simulink model "single_module"  (R2018a)
settings: Solver=FixedStepDiscrete  StartTime=0.0  StopTime=Tfinal  FixedStep=SampleTime  RelTol=1e-3
values from neighbouring files (symbols this model uses):
  C1A = 5e-6    (= 5e-06)    [capacitor_A.m]    (also in impedance_phA.m; param_single_module_parasitic.m; trial_capacitor_response.m)
  C1B = 5e-6    (= 5e-06)    [capacitor_A.m]    (also in impedance_phA.m; param_single_module_parasitic.m; trial_capacitor_response.m)
  C1C = 5e-6    (= 5e-06)    [capacitor_A.m]    (also in impedance_phA.m; param_single_module_parasitic.m; trial_capacitor_response.m)
  ESLA = 19e-9    (= 1.9e-08)    [capacitor_A.m]    (also in impedance_phA.m; param_single_module_parasitic.m; trial_capacitor_response.m)
  ESLB = 19e-9    (= 1.9e-08)    [capacitor_A.m]    (also in impedance_phA.m; param_single_module_parasitic.m; trial_capacitor_response.m)
  ESLC = 19e-9    (= 1.9e-08)    [capacitor_A.m]    (also in impedance_phA.m; param_single_module_parasitic.m; trial_capacitor_response.m)
  ESRA = 21.1e-3    (= 0.0211)    [impedance_phA.m]    (also in param_single_module_parasitic.m)
  ESRB = 21.1e-3    (= 0.0211)    [impedance_phA.m]    (also in param_single_module_parasitic.m)
  ESRC = 21.1e-3    (= 0.0211)    [impedance_phA.m]    (also in param_single_module_parasitic.m)
  ffund = 50    [param_single_module_parasitic.m]
  LABBot = 10.20e-9    (= 1.02e-08)    [capacitor_A.m]    (also in impedance_phA.m; param_single_module_parasitic.m; trial_capacitor_response.m)
  LABot = 20.25e-9    (= 2.025e-08)    [capacitor_A.m]    (also in impedance_phA.m; param_single_module_parasitic.m; trial_capacitor_response.m)
  LABTop = 18.30e-9    (= 1.83e-08)    [capacitor_A.m]    (also in impedance_phA.m; param_single_module_parasitic.m; trial_capacitor_response.m)
  LAMid = 01.30e-9    (= 1.3e-09)    [capacitor_A.m]    (also in impedance_phA.m; param_single_module_parasitic.m; trial_capacitor_response.m)
  LATop = 03.40e-9    (= 3.4e-09)    [capacitor_A.m]    (also in impedance_phA.m; param_single_module_parasitic.m; trial_capacitor_response.m)
  LBBot = 20.38e-9    (= 2.038e-08)    [capacitor_A.m]    (also in impedance_phA.m; param_single_module_parasitic.m; trial_capacitor_response.m)
  LBCBot = 11.14e-9    (= 1.114e-08)    [capacitor_A.m]    (also in impedance_phA.m; param_single_module_parasitic.m; trial_capacitor_response.m)
  LBCTop = 21.84e-9    (= 2.184e-08)    [capacitor_A.m]    (also in impedance_phA.m; param_single_module_parasitic.m; trial_capacitor_response.m)
  LBMid = 01.30e-9    (= 1.3e-09)    [capacitor_A.m]    (also in impedance_phA.m; param_single_module_parasitic.m; trial_capacitor_response.m)
  LBTop = 03.38e-9    (= 3.38e-09)    [capacitor_A.m]    (also in impedance_phA.m; param_single_module_parasitic.m; trial_capacitor_response.m)
  LCBot = 20.94e-9    (= 2.094e-08)    [capacitor_A.m]    (also in impedance_phA.m; param_single_module_parasitic.m; trial_capacitor_response.m)
  LCMid = 01.30e-9    (= 1.3e-09)    [capacitor_A.m]    (also in impedance_phA.m; param_single_module_parasitic.m; trial_capacitor_response.m)
  LCTop = 03.41e-9    (= 3.41e-09)    [capacitor_A.m]    (also in impedance_phA.m; param_single_module_parasitic.m; trial_capacitor_response.m)
  Lin = 1e-4    (= 0.0001)    [capacitor_A.m]    (also in impedance_phA.m = 1e-06; param_single_module_parasitic.m = 1e-06; trial_capacitor_response.m)
  Lload1 = Xload1/(2*pi*ffund)    [param_single_module_parasitic.m]
  ModulationIndex1 = 0.9    [param_single_module_parasitic.m]
  Module1Phase = 0    [param_single_module_parasitic.m]
  Rin = 20    [capacitor_A.m]    (also in impedance_phA.m = 0.1; param_single_module_parasitic.m = 0.1; trial_capacitor_response.m = 50)
  Rload1 = Z1*PF    [param_single_module_parasitic.m]
  SampleTime = 1e-8    (= 1e-08)    [param_single_module_parasitic.m]
  Vin = Vdc + Idc*Rin    (= 270.740740741)    [param_single_module_parasitic.m]
libraries: powerlib x45, simulink x6, powerlib_meascontrol x1
settings Model: Creator=enes_  LastModifiedBy=enes_

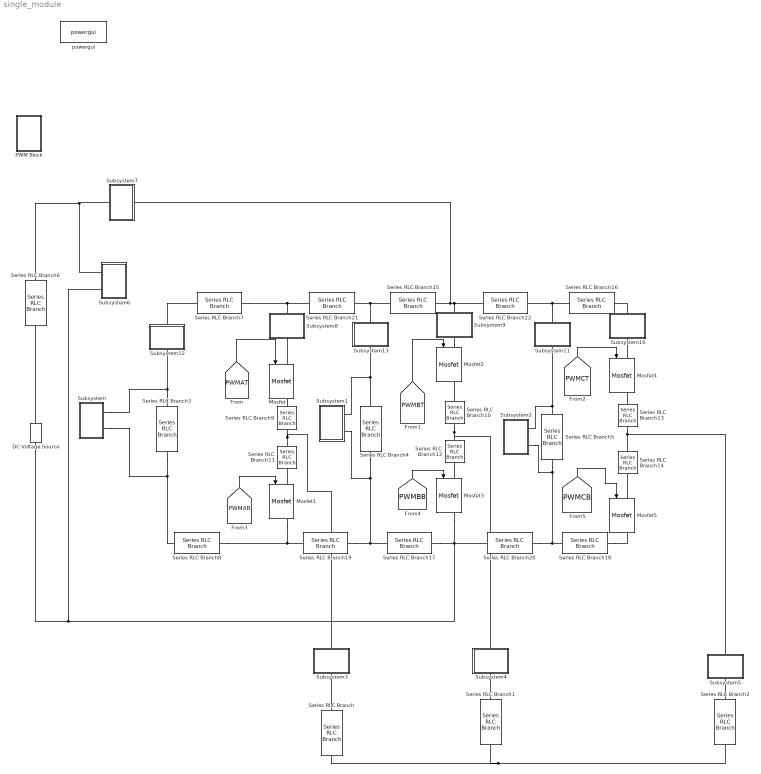
== system single_module ==
  DC Voltage Source : powerlib/Electrical Sources/DC Voltage Source  Amplitude=Vin  Measurements=None
  Mosfet{,1..5} (6 alike) : powerlib/Power Electronics/Mosfet  Ron=0.1  Lon=0  Rd=0.01  Vfd=0  IC=0  Rs=1e5  Cs=inf  Measurements=on
  PWM Block : Subsystem
  Series RLC Branch : powerlib/Elements/Series RLC Branch  LConnTagsString=__new0  RConnTagsString=__new0  BranchType=RL  Resistance=Rload1  Inductance=Lload1  SetiL0=off  InitialCurrent=0  Capacitance=1e-6  Setx0=off  InitialVoltage=0  Measurements=None
  Series RLC Branch1 : powerlib/Elements/Series RLC Branch  LConnTagsString=__new0  RConnTagsString=__new0  BranchType=RL  Resistance=Rload1  Inductance=Lload1  SetiL0=off  InitialCurrent=0  Capacitance=1e-6  Setx0=off  InitialVoltage=0  Measurements=None
  Series RLC Branch10 : powerlib/Elements/Series RLC Branch  LConnTagsString=__new0  RConnTagsString=__new0  BranchType=L  Resistance=1  Inductance=LBMid/2  SetiL0=off  InitialCurrent=0  Capacitance=1e-6  Setx0=off  InitialVoltage=0  Measurements=None
  Series RLC Branch11 : powerlib/Elements/Series RLC Branch  LConnTagsString=__new0  RConnTagsString=__new0  BranchType=L  Resistance=1  Inductance=LAMid/2  SetiL0=off  InitialCurrent=0  Capacitance=1e-6  Setx0=off  InitialVoltage=0  Measurements=None
  Series RLC Branch12 : powerlib/Elements/Series RLC Branch  LConnTagsString=__new0  RConnTagsString=__new0  BranchType=L  Resistance=1  Inductance=LBMid/2  SetiL0=off  InitialCurrent=0  Capacitance=1e-6  Setx0=off  InitialVoltage=0  Measurements=None
  Series RLC Branch13 : powerlib/Elements/Series RLC Branch  LConnTagsString=__new0  RConnTagsString=__new0  BranchType=L  Resistance=1  Inductance=LCMid/2  SetiL0=off  InitialCurrent=0  Capacitance=1e-6  Setx0=off  InitialVoltage=0  Measurements=None
  Series RLC Branch14 : powerlib/Elements/Series RLC Branch  LConnTagsString=__new0  RConnTagsString=__new0  BranchType=L  Resistance=1  Inductance=LCMid/2  SetiL0=off  InitialCurrent=0  Capacitance=1e-6  Setx0=off  InitialVoltage=0  Measurements=None
  Series RLC Branch15 : powerlib/Elements/Series RLC Branch  LConnTagsString=__new0  RConnTagsString=__new0  BranchType=L  Resistance=1  Inductance=LBTop  SetiL0=off  InitialCurrent=0  Capacitance=1e-6  Setx0=off  InitialVoltage=0  Measurements=None
  Series RLC Branch16 : powerlib/Elements/Series RLC Branch  LConnTagsString=__new0  RConnTagsString=__new0  BranchType=L  Resistance=1  Inductance=LCTop  SetiL0=off  InitialCurrent=0  Capacitance=1e-6  Setx0=off  InitialVoltage=0  Measurements=None
  Series RLC Branch17 : powerlib/Elements/Series RLC Branch  LConnTagsString=__new0  RConnTagsString=__new0  BranchType=L  Resistance=1  Inductance=LBBot  SetiL0=off  InitialCurrent=0  Capacitance=1e-6  Setx0=off  InitialVoltage=0  Measurements=None
  Series RLC Branch18 : powerlib/Elements/Series RLC Branch  LConnTagsString=__new0  RConnTagsString=__new0  BranchType=L  Resistance=1  Inductance=LCBot  SetiL0=off  InitialCurrent=0  Capacitance=1e-6  Setx0=off  InitialVoltage=0  Measurements=None
  Series RLC Branch19 : powerlib/Elements/Series RLC Branch  LConnTagsString=__new0  RConnTagsString=__new0  BranchType=L  Resistance=1  Inductance=LABBot  SetiL0=off  InitialCurrent=0  Capacitance=1e-6  Setx0=off  InitialVoltage=0  Measurements=None
  Series RLC Branch2 : powerlib/Elements/Series RLC Branch  LConnTagsString=__new0  RConnTagsString=__new0  BranchType=RL  Resistance=Rload1  Inductance=Lload1  SetiL0=off  InitialCurrent=0  Capacitance=1e-6  Setx0=off  InitialVoltage=0  Measurements=None
  Series RLC Branch20 : powerlib/Elements/Series RLC Branch  LConnTagsString=__new0  RConnTagsString=__new0  BranchType=L  Resistance=1  Inductance=LBCBot  SetiL0=off  InitialCurrent=0  Capacitance=1e-6  Setx0=off  InitialVoltage=0  Measurements=None
  Series RLC Branch21 : powerlib/Elements/Series RLC Branch  LConnTagsString=__new0  RConnTagsString=__new0  BranchType=L  Resistance=1  Inductance=LABTop  SetiL0=off  InitialCurrent=0  Capacitance=1e-6  Setx0=off  InitialVoltage=0  Measurements=None
  Series RLC Branch22 : powerlib/Elements/Series RLC Branch  LConnTagsString=__new0  RConnTagsString=__new0  BranchType=L  Resistance=1  Inductance=LBCTop  SetiL0=off  InitialCurrent=0  Capacitance=1e-6  Setx0=off  InitialVoltage=0  Measurements=None
  Series RLC Branch3 : powerlib/Elements/Series RLC Branch  LConnTagsString=__new0  RConnTagsString=__new0  BranchType=RLC  Resistance=ESRA  Inductance=ESLA  SetiL0=off  InitialCurrent=0  Capacitance=C1A  Setx0=off  InitialVoltage=0  Measurements=None
  Series RLC Branch4 : powerlib/Elements/Series RLC Branch  LConnTagsString=__new0  RConnTagsString=__new0  BranchType=RLC  Resistance=ESRB  Inductance=ESLB  SetiL0=off  InitialCurrent=0  Capacitance=C1B  Setx0=off  InitialVoltage=0  Measurements=None
  Series RLC Branch5 : powerlib/Elements/Series RLC Branch  LConnTagsString=__new0  RConnTagsString=__new0  BranchType=RLC  Resistance=ESRC  Inductance=ESLC  SetiL0=off  InitialCurrent=0  Capacitance=C1C  Setx0=off  InitialVoltage=0  Measurements=None
  Series RLC Branch6 : powerlib/Elements/Series RLC Branch  LConnTagsString=__new0  RConnTagsString=__new0  BranchType=RL  Resistance=Rin  Inductance=Lin  SetiL0=off  InitialCurrent=0  Capacitance=C1A  Setx0=off  InitialVoltage=0  Measurements=None
  Series RLC Branch7 : powerlib/Elements/Series RLC Branch  LConnTagsString=__new0  RConnTagsString=__new0  BranchType=L  Resistance=1  Inductance=LATop  SetiL0=off  InitialCurrent=0  Capacitance=1e-6  Setx0=off  InitialVoltage=0  Measurements=None
  Series RLC Branch8 : powerlib/Elements/Series RLC Branch  LConnTagsString=__new0  RConnTagsString=__new0  BranchType=L  Resistance=1  Inductance=LABot  SetiL0=off  InitialCurrent=0  Capacitance=1e-6  Setx0=off  InitialVoltage=0  Measurements=None
  Series RLC Branch9 : powerlib/Elements/Series RLC Branch  LConnTagsString=__new0  RConnTagsString=__new0  BranchType=L  Resistance=1  Inductance=LAMid/2  SetiL0=off  InitialCurrent=0  Capacitance=1e-6  Setx0=off  InitialVoltage=0  Measurements=None
  Subsystem : Subsystem
  Subsystem1 : Subsystem
  Subsystem10 : Subsystem
  Subsystem11 : Subsystem
  Subsystem12 : Subsystem
  Subsystem13 : Subsystem
  Subsystem2 : Subsystem
  Subsystem3 : Subsystem
  Subsystem4 : Subsystem
  Subsystem5 : Subsystem
  Subsystem6 : Subsystem
  Subsystem7 : Subsystem
  Subsystem8 : Subsystem
  Subsystem9 : Subsystem
  powergui : powerlib/powergui  Priority=1  SimulationMode=Discrete  SampleTime=SampleTime  frequency=60  Iterations=50  frequencyindice=0  Pbase=100e6  ErrMax=1e-4  UnitsV=kV  UnitsW=MW  buscounter=0  FunctionMessages=off  echomessages=off  EnableUseOfTLC=off  CurrentSourceSwitches=off  DisableSnubberDevices=off  DisableRonSwitches=off  DisableVfSwitches=off  DisplayEquations=off  SolverType=Tustin/Backward Euler (TBE)  Interpol=off  ExternalGateDelay=off  methode=off  Ts=100  x0status=blocks  SPID=on  SwTol=0  HookPort=off  RestoreLinks=warning  ResistiveCurrentMeasurement=off  Frange=[0:2:500]  Ylog=off  Xlog=on  ShowGrid=off  save=off  variable=ZData  structure=0  ZoomFFT=off  StartTime=0.0  cycles=1  DisplayStyle=1  fundamental=60  FreqAxis=off  MaxFrequency=1000  frequencyindicesteady=1  RmsSteady=1  display=off
  wires:
  [PWMAT] -> Mosfet/1
  [PWMAB] -> Mosfet1/1
  [PWMBB] -> Mosfet3/1
  [PWMBT] -> Mosfet2/1
  [PWMCB] -> Mosfet5/1
  [PWMCT] -> Mosfet4/1
  connections:
  Subsystem10/RConn1 -- Series RLC Branch16/RConn1
  Series RLC Branch17/LConn1 -- Subsystem1/LConn2 -- Series RLC Branch4/RConn1 -- Series RLC Branch19/RConn1
  Mosfet1/LConn1 -- Series RLC Branch11/RConn1
  Mosfet3/LConn1 -- Series RLC Branch12/RConn1
  Series RLC Branch13/RConn1 -- Series RLC Branch14/LConn1 -- Subsystem5/RConn1
  Series RLC Branch/RConn1 -- Series RLC Branch2/RConn1 -- Series RLC Branch1/RConn1
  DC Voltage Source/RConn1 -- Series RLC Branch6/RConn1
  Series RLC Branch/LConn1 -- Subsystem3/LConn1
  Series RLC Branch1/LConn1 -- Subsystem4/LConn1
  Series RLC Branch2/LConn1 -- Subsystem5/LConn1
  Subsystem6/LConn1 -- Subsystem7/RConn1 -- Series RLC Branch6/LConn1
  Mosfet/LConn1 -- Subsystem8/LConn1
  Subsystem9/LConn1 -- Mosfet2/LConn1
  Mosfet4/LConn1 -- Subsystem10/LConn1
  Subsystem2/LConn1 -- Series RLC Branch5/LConn1 -- Subsystem11/LConn1
  Subsystem/LConn1 -- Subsystem12/LConn1 -- Series RLC Branch3/LConn1
  Subsystem1/LConn1 -- Subsystem13/LConn1 -- Series RLC Branch4/LConn1
  Subsystem12/RConn1 -- Series RLC Branch7/LConn1
  Subsystem/LConn2 -- Series RLC Branch8/LConn1 -- Series RLC Branch3/RConn1
  Series RLC Branch9/LConn1 -- Mosfet/RConn1
  Series RLC Branch11/LConn1 -- Subsystem3/RConn1 -- Series RLC Branch9/RConn1
  Series RLC Branch10/LConn1 -- Mosfet2/RConn1
  Series RLC Branch12/LConn1 -- Subsystem4/RConn1 -- Series RLC Branch10/RConn1
  Series RLC Branch13/LConn1 -- Mosfet4/RConn1
  Mosfet5/LConn1 -- Series RLC Branch14/RConn1
  Series RLC Branch15/LConn1 -- Subsystem13/RConn1 -- Series RLC Branch21/RConn1
  Subsystem7/LConn1 -- Series RLC Branch22/LConn1 -- Subsystem9/RConn1 -- Series RLC Branch15/RConn1
  Series RLC Branch17/RConn1 -- Mosfet3/RConn1 -- Series RLC Branch20/LConn1 -- Subsystem6/LConn2 -- DC Voltage Source/LConn1
  Series RLC Branch18/RConn1 -- Mosfet5/RConn1
  Series RLC Branch8/RConn1 -- Mosfet1/RConn1 -- Series RLC Branch19/LConn1
  Series RLC Branch5/RConn1 -- Subsystem2/LConn2 -- Series RLC Branch20/RConn1 -- Series RLC Branch18/LConn1
  Series RLC Branch21/LConn1 -- Subsystem8/RConn1 -- Series RLC Branch7/RConn1
  Series RLC Branch16/LConn1 -- Subsystem11/RConn1 -- Series RLC Branch22/RConn1

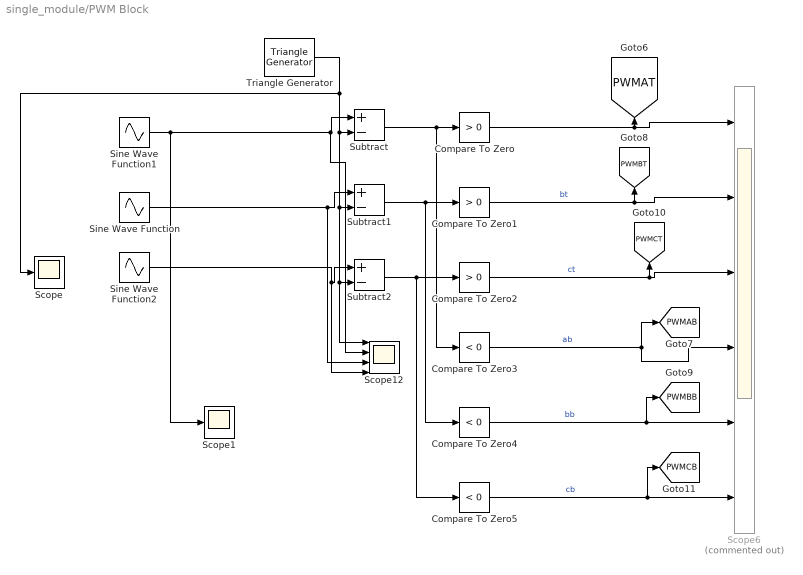
== system single_module/PWM Block ==
  Compare To Zero : simulink/Logic and Bit Operations/Compare To Zero  relop=>  OutDataTypeStr=boolean
  Compare To Zero1 : simulink/Logic and Bit Operations/Compare To Zero  relop=>  OutDataTypeStr=boolean
  Compare To Zero2 : simulink/Logic and Bit Operations/Compare To Zero  relop=>  OutDataTypeStr=boolean
  Compare To Zero3 : simulink/Logic and Bit Operations/Compare To Zero  relop=<  OutDataTypeStr=boolean
  Compare To Zero4 : simulink/Logic and Bit Operations/Compare To Zero  relop=<  OutDataTypeStr=boolean
  Compare To Zero5 : simulink/Logic and Bit Operations/Compare To Zero  relop=<  OutDataTypeStr=boolean
  Scope : Scope
  Scope1 : Scope
  Scope12 : Scope  NumInputPorts=4
  Scope6 : Scope  Commented=on  NumInputPorts=6
  Sine Wave Function : Sin  Amplitude=ModulationIndex1  Frequency=ffund*2*pi  Phase=-2*pi/3  SampleTime=0
  Sine Wave Function1 : Sin  Amplitude=ModulationIndex1  Frequency=ffund*2*pi  SampleTime=0
  Sine Wave Function2 : Sin  Amplitude=ModulationIndex1  Frequency=ffund*2*pi  Phase=2*pi/3  SampleTime=0
  Subtract : Sum  Inputs=+-
  Subtract1 : Sum  Inputs=+-
  Subtract2 : Sum  Inputs=+-
  Triangle Generator : powerlib_meascontrol/Pulse & Signal Generators/Triangle Generator  Freq=fsw  Phase=Module1Phase  Ts=0
  tag scope: PWMAB=global, PWMAT=global, PWMBB=global, PWMBT=global, PWMCB=global, PWMCT=global
  wires:
  Compare To Zero2/1 -> [PWMCT], Scope6/3  "ct"
  Sine Wave Function/1 -> Subtract1/1, Scope12/3
  Subtract2/1 -> Compare To Zero5/1, Compare To Zero2/1
  Sine Wave Function1/1 -> Scope1/1, Scope12/2, Subtract/1
  Subtract1/1 -> Compare To Zero4/1, Compare To Zero1/1
  Triangle Generator/1 -> Scope/1, Scope12/1, Subtract2/2, Subtract1/2, Subtract/2
  Compare To Zero/1 -> Scope6/1, [PWMAT]
  Subtract/1 -> Compare To Zero3/1, Compare To Zero/1
  Compare To Zero1/1 -> [PWMBT], Scope6/2  "bt"
  Compare To Zero5/1 -> [PWMCB], Scope6/6  "cb"
  Compare To Zero4/1 -> [PWMBB], Scope6/5  "bb"
  Sine Wave Function2/1 -> Scope12/4, Subtract2/1
  Compare To Zero3/1 -> [PWMAB], Scope6/4  "ab"

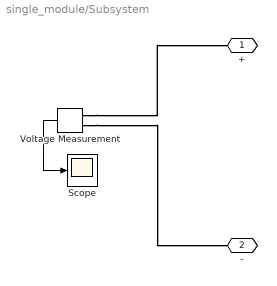
== system single_module/Subsystem ==
  Scope : Scope
  Voltage Measurement : powerlib/Measurements/Voltage Measurement  PhasorSimulation=off  OutputType=Complex  PSBequivalent=0
  + : PMIOPort  Side=Left
  - : PMIOPort  Port=2  Side=Left
  wires:
  Voltage Measurement/1 -> Scope/1
  connections:
  Voltage Measurement/LConn1 -- +/RConn1
  Voltage Measurement/LConn2 -- -/RConn1

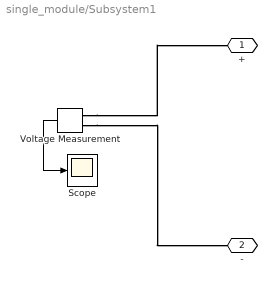
== system single_module/Subsystem1 ==
  Scope : Scope
  Voltage Measurement : powerlib/Measurements/Voltage Measurement  PhasorSimulation=off  OutputType=Complex  PSBequivalent=0
  + : PMIOPort  Side=Left
  - : PMIOPort  Port=2  Side=Left
  wires:
  Voltage Measurement/1 -> Scope/1
  connections:
  Voltage Measurement/LConn1 -- +/RConn1
  Voltage Measurement/LConn2 -- -/RConn1

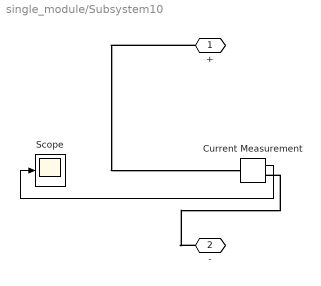
== system single_module/Subsystem10 ==
  Current Measurement : powerlib/Measurements/Current Measurement  PhasorSimulation=off  OutputType=Complex  PSBequivalent=0
  Scope : Scope
  + : PMIOPort  Side=Right
  - : PMIOPort  Port=2  Side=Left
  wires:
  Current Measurement/1 -> Scope/1
  connections:
  +/RConn1 -- Current Measurement/LConn1
  -/RConn1 -- Current Measurement/RConn1

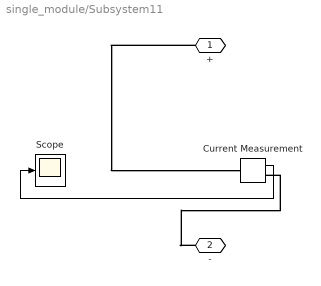
== system single_module/Subsystem11 ==
  Current Measurement : powerlib/Measurements/Current Measurement  PhasorSimulation=off  OutputType=Complex  PSBequivalent=0
  Scope : Scope
  + : PMIOPort  Side=Right
  - : PMIOPort  Port=2  Side=Left
  wires:
  Current Measurement/1 -> Scope/1
  connections:
  +/RConn1 -- Current Measurement/LConn1
  -/RConn1 -- Current Measurement/RConn1

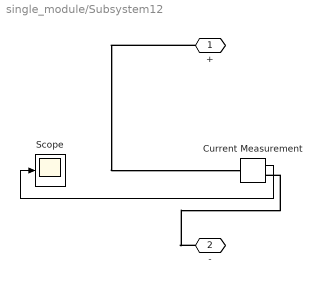
== system single_module/Subsystem12 ==
  Current Measurement : powerlib/Measurements/Current Measurement  PhasorSimulation=off  OutputType=Complex  PSBequivalent=0
  Scope : Scope
  + : PMIOPort  Side=Right
  - : PMIOPort  Port=2  Side=Left
  wires:
  Current Measurement/1 -> Scope/1
  connections:
  +/RConn1 -- Current Measurement/LConn1
  -/RConn1 -- Current Measurement/RConn1

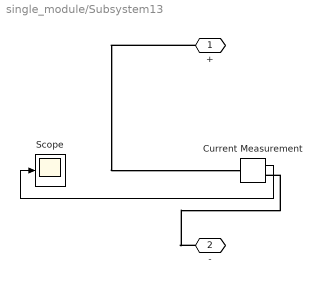
== system single_module/Subsystem13 ==
  Current Measurement : powerlib/Measurements/Current Measurement  PhasorSimulation=off  OutputType=Complex  PSBequivalent=0
  Scope : Scope
  + : PMIOPort  Side=Right
  - : PMIOPort  Port=2  Side=Left
  wires:
  Current Measurement/1 -> Scope/1
  connections:
  +/RConn1 -- Current Measurement/LConn1
  -/RConn1 -- Current Measurement/RConn1

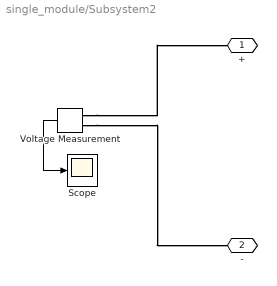
== system single_module/Subsystem2 ==
  Scope : Scope
  Voltage Measurement : powerlib/Measurements/Voltage Measurement  PhasorSimulation=off  OutputType=Complex  PSBequivalent=0
  + : PMIOPort  Side=Left
  - : PMIOPort  Port=2  Side=Left
  wires:
  Voltage Measurement/1 -> Scope/1
  connections:
  Voltage Measurement/LConn1 -- +/RConn1
  Voltage Measurement/LConn2 -- -/RConn1

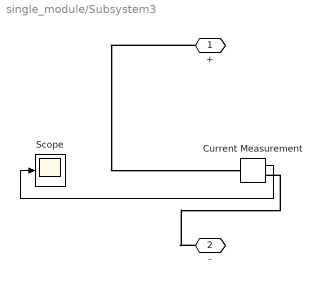
== system single_module/Subsystem3 ==
  Current Measurement : powerlib/Measurements/Current Measurement  PhasorSimulation=off  OutputType=Complex  PSBequivalent=0
  Scope : Scope
  + : PMIOPort  Side=Right
  - : PMIOPort  Port=2  Side=Left
  wires:
  Current Measurement/1 -> Scope/1
  connections:
  +/RConn1 -- Current Measurement/LConn1
  -/RConn1 -- Current Measurement/RConn1

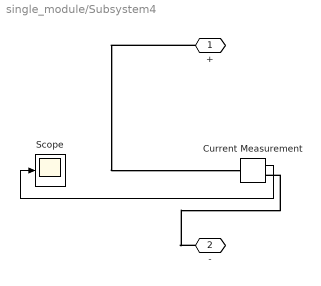
== system single_module/Subsystem4 ==
  Current Measurement : powerlib/Measurements/Current Measurement  PhasorSimulation=off  OutputType=Complex  PSBequivalent=0
  Scope : Scope
  + : PMIOPort  Side=Right
  - : PMIOPort  Port=2  Side=Left
  wires:
  Current Measurement/1 -> Scope/1
  connections:
  +/RConn1 -- Current Measurement/LConn1
  -/RConn1 -- Current Measurement/RConn1

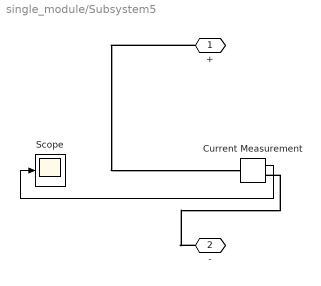
== system single_module/Subsystem5 ==
  Current Measurement : powerlib/Measurements/Current Measurement  PhasorSimulation=off  OutputType=Complex  PSBequivalent=0
  Scope : Scope
  + : PMIOPort  Side=Right
  - : PMIOPort  Port=2  Side=Left
  wires:
  Current Measurement/1 -> Scope/1
  connections:
  +/RConn1 -- Current Measurement/LConn1
  -/RConn1 -- Current Measurement/RConn1

== system single_module/Subsystem6 ==
  Scope : Scope
  Voltage Measurement : powerlib/Measurements/Voltage Measurement  PhasorSimulation=off  OutputType=Complex  PSBequivalent=0
  + : PMIOPort  Side=Left
  - : PMIOPort  Port=2  Side=Left
  wires:
  Voltage Measurement/1 -> Scope/1
  connections:
  Voltage Measurement/LConn1 -- +/RConn1
  Voltage Measurement/LConn2 -- -/RConn1

== system single_module/Subsystem7 ==
  Current Measurement : powerlib/Measurements/Current Measurement  PhasorSimulation=off  OutputType=Complex  PSBequivalent=0
  Scope : Scope
  + : PMIOPort  Side=Right
  - : PMIOPort  Port=2  Side=Left
  wires:
  Current Measurement/1 -> Scope/1
  connections:
  +/RConn1 -- Current Measurement/LConn1
  -/RConn1 -- Current Measurement/RConn1

== system single_module/Subsystem8 ==
  Current Measurement : powerlib/Measurements/Current Measurement  PhasorSimulation=off  OutputType=Complex  PSBequivalent=0
  Scope : Scope
  + : PMIOPort  Side=Right
  - : PMIOPort  Port=2  Side=Left
  wires:
  Current Measurement/1 -> Scope/1
  connections:
  +/RConn1 -- Current Measurement/LConn1
  -/RConn1 -- Current Measurement/RConn1

== system single_module/Subsystem9 ==
  Current Measurement : powerlib/Measurements/Current Measurement  PhasorSimulation=off  OutputType=Complex  PSBequivalent=0
  Scope : Scope
  + : PMIOPort  Side=Right
  - : PMIOPort  Port=2  Side=Left
  wires:
  Current Measurement/1 -> Scope/1
  connections:
  +/RConn1 -- Current Measurement/LConn1
  -/RConn1 -- Current Measurement/RConn1
